simulink model "P_Like"  (Simulink 7.3)
settings: Solver=ode45  StartTime=0.0  StopTime=100  RelTol=1e-3
values from neighbouring files (symbols this model uses):
  Dm = 0.2    [Parameters.m]
  Ds = 0.1    [Parameters.m]
  K = ceil(max(K1,K2))    [Gains.m]
  Lm1 = 0.5    [Parameters.m]
  Lm2 = 0.5    [Parameters.m]
  Ls1 = 0.5    [Parameters.m]
  Ls2 = 0.5    [Parameters.m]
  Mm1 = 1    [Parameters.m]
  Mm2 = 1    [Parameters.m]
  Ms1 = 2    [Parameters.m]
  Ms2 = 2    [Parameters.m]
  P = 10    [Parameters.m]
  q0 = [0;0]    [Parameters.m]
  v0 = [0;0;0]    [Initiation.m]    (also in Parameters.m = [0;0])
settings Model: Creator=TOSHIBA  LastModifiedBy=TOSHIBA  CovModelRefEnable=off
settings DataIOCC: SaveFormat=StructureWithTime  ReturnWorkspaceOutputs=off
settings OptimizationCC: ExpressionDepthLimit=128
settings DebuggingCC: UnderspecifiedInitializationDetection=Simplified  MergeDetectMultiDrivingBlocksExec=error  SolverPrmCheckMsg=none  FcnCallInpInsideContextMsg=Enable All  StateNameClashWarn=none  StrictBusMsg=ErrorLevel1
settings HardwareCC: ProdIntDivRoundTo=Zero  ProdEndianess=LittleEndian  ProdHWDeviceType=Specified
settings CodeAppCC: CustomSymbolStrType=$N$R$M_T
settings GRTTargetCC: TargetFunctionLibrary=C89/C90 (ANSI)

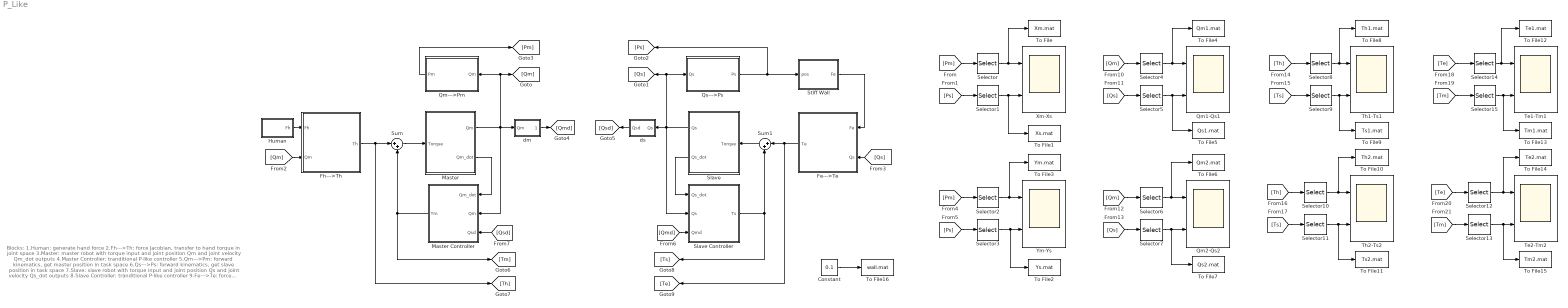
== system P_Like ==
  note: Blocks:
      | 1.Human: generate hand force
      | 2.Fh--->Th: force Jacobian, transfer to hand torque in joint space
      | 3.Master: master robot with torque input and joint position Qm and joint velocity Qm_dot outputs
      | 4.Master Controller: tranditional P-like controller
      | 5.Qm--->Pm: forward kinematics, get master position in task space
      | 6.Qs--->Ps: forward kinematics, get slave position in task space
      | 7.Slave: slave robot with torque input and joint position Qs and joint velocity Qs_dot outputs
      | 8.Slave Controller: tranditional P-like controller
      | 9.Fe--->Te: force Jacobian, transfer to environment torque in joint space
      | 10.Stiff Wall: spring with k=10KN/m
  Constant : Constant  Value=0.1
  Fe--->Te : Subsystem
  Fh--->Th : Subsystem
  Human : Subsystem
  Master : Subsystem
  Master Controller : Subsystem
  Qm--->Pm : Subsystem
  Qm1-Qs1 : Scope  NumInputPorts=2
      settings: TimeRange=auto  MaxDataPoints=5000  SaveToWorkspace=off  SaveName=ScopeData2  YMin=-0.1601~-5  YMax=0.25682~5  SampleTime=-1
  Qm2-Qs2 : Scope  NumInputPorts=2
      settings: TimeRange=auto  MaxDataPoints=5000  SaveToWorkspace=off  SaveName=ScopeData3  YMin=-0.08778~-5  YMax=0.12467~5  SampleTime=-1
  Qs--->Ps : Subsystem
  Selector{,1,4..5,8..9,14..15} (8 alike) : Selector  InputPortWidth=2  IndexOptions=Index vector (dialog)  Indices=[1]  OutputSizes=1
  Selector{2..3,6..7,10..13} (8 alike) : Selector  InputPortWidth=2  IndexOptions=Index vector (dialog)  Indices=[2]  OutputSizes=1
  Slave : Subsystem
  Slave Controller : Subsystem
  Stiff Wall : Stateflow chart  TreatAsAtomicUnit=on
      settings: PermitHierarchicalResolution=ParametersOnly
  Sum : Sum  Inputs=|++
  Sum1 : Sum  Inputs=|++
  Te1-Tm1 : Scope  NumInputPorts=2
      settings: TimeRange=auto  MaxDataPoints=5000  SaveToWorkspace=off  SaveName=ScopeData6  YMin=-10.54121~-5  YMax=1.73671~5  SampleTime=-1
  Te2-Tm2 : Scope  NumInputPorts=2
      settings: TimeRange=auto  MaxDataPoints=5000  SaveToWorkspace=off  SaveName=ScopeData7  YMin=-5.26164~-5  YMax=0.8676~5  SampleTime=-1
  Th1-Ts1 : Scope  NumInputPorts=2
      settings: TimeRange=auto  MaxDataPoints=5000  SaveToWorkspace=off  SaveName=ScopeData4  YMin=-0.80713~-5  YMax=2.31036~5  SampleTime=-1
  Th2-Ts2 : Scope  NumInputPorts=2
      settings: TimeRange=auto  MaxDataPoints=5000  SaveToWorkspace=off  SaveName=ScopeData5  YMin=-0.4004~-5  YMax=1.10559~5  SampleTime=-1
  To File : ToFile  Filename=Xm.mat  MatrixName=Xm
  To File1 : ToFile  Filename=Xs.mat  MatrixName=Xs
  To File10 : ToFile  Filename=Th2.mat  MatrixName=Th2
  To File11 : ToFile  Filename=Ts2.mat  MatrixName=Ts2
  To File12 : ToFile  Filename=Te1.mat  MatrixName=Te1
  To File13 : ToFile  Filename=Tm1.mat  MatrixName=Tm1
  To File14 : ToFile  Filename=Te2.mat  MatrixName=Te2
  To File15 : ToFile  Filename=Tm2.mat  MatrixName=Tm2
  To File16 : ToFile  Filename=wall.mat  MatrixName=wall
  To File2 : ToFile  Filename=Ys.mat  MatrixName=Ys
  To File3 : ToFile  Filename=Ym.mat  MatrixName=Ym
  To File4 : ToFile  Filename=Qm1.mat  MatrixName=Qm1
  To File5 : ToFile  Filename=Qs1.mat  MatrixName=Qs1
  To File6 : ToFile  Filename=Qm2.mat  MatrixName=Qm2
  To File7 : ToFile  Filename=Qs2.mat  MatrixName=Qs2
  To File8 : ToFile  Filename=Th1.mat  MatrixName=Th1
  To File9 : ToFile  Filename=Ts1.mat  MatrixName=Ts1
  Xm-Xs : Scope  NumInputPorts=2
      settings: TimeRange=auto  MaxDataPoints=5000  SaveToWorkspace=off  SaveName=ScopeData  YMin=0.95971~-5  YMax=1.00448~5  SampleTime=-1
  Ym-Ys : Scope  NumInputPorts=2
      settings: TimeRange=auto  MaxDataPoints=5000  SaveToWorkspace=off  YMin=-0.20079~-5  YMax=0.31146~5  SampleTime=-1
  dm : Subsystem
  ds : Subsystem
  wires:
  Qs--->Ps/1(Ps) -> [Ps], Stiff Wall/1(pos)
  Stiff Wall/1(Fe) -> Fe--->Te/1(Fe)
  Fe--->Te/1(Te) -> Sum1/1, [Te]
  Sum1/1 -> Slave/1(Torque)
  Sum/1 -> Master/1(Torque)
  Fh--->Th/1(Th) -> [Th], Sum/1
  Master/2(Qm_dot) -> Master Controller/1(Qm_dot)
  Master Controller/1(Tm) -> Sum/2, [Tm]
  Slave/2(Qs_dot) -> Slave Controller/1(Qs_dot)
  Slave Controller/1(Ts) -> [Ts], Sum1/2
  [Qs] -> Fe--->Te/2(Qs)
  Master/1(Qm) -> dm/1(Qm), Qm--->Pm/1(Qm), [Qm], Master Controller/2(Qm)
  Slave/1(Qs) -> ds/1(Qs), [Qs], Qs--->Ps/1(Qs), Slave Controller/2(Qs)
  [Qm] -> Fh--->Th/2(Qm)
  Human/1(Fh) -> Fh--->Th/1(Fh)
  Qm--->Pm/1(Pm) -> [Pm]
  [Pm] -> Selector/1
  Selector/1 -> To File/1, Xm-Xs/1
  [Ps] -> Selector1/1
  Selector1/1 -> To File1/1, Xm-Xs/2
  [Pm] -> Selector2/1
  Selector2/1 -> To File3/1, Ym-Ys/1
  [Ps] -> Selector3/1
  Selector3/1 -> To File2/1, Ym-Ys/2
  [Qmd] -> Slave Controller/3(Qmd)
  dm/1(Qmd) -> [Qmd]
  ds/1(Qsd) -> [Qsd]
  [Qsd] -> Master Controller/3(Qsd)
  [Qs] -> Selector5/1
  [Qm] -> Selector4/1
  Selector4/1 -> To File4/1, Qm1-Qs1/1
  Selector5/1 -> To File5/1, Qm1-Qs1/2
  [Qs] -> Selector7/1
  [Qm] -> Selector6/1
  Selector6/1 -> To File6/1, Qm2-Qs2/1
  Selector7/1 -> To File7/1, Qm2-Qs2/2
  [Th] -> Selector8/1
  [Ts] -> Selector9/1
  Selector9/1 -> To File9/1, Th1-Ts1/2
  Selector8/1 -> To File8/1, Th1-Ts1/1
  [Ts] -> Selector11/1
  [Th] -> Selector10/1
  Selector10/1 -> To File10/1, Th2-Ts2/1
  [Te] -> Selector14/1
  [Tm] -> Selector15/1
  Selector15/1 -> To File13/1, Te1-Tm1/2
  Selector14/1 -> To File12/1, Te1-Tm1/1
  [Tm] -> Selector13/1
  [Te] -> Selector12/1
  Selector12/1 -> To File14/1, Te2-Tm2/1
  Selector13/1 -> To File15/1, Te2-Tm2/2
  Selector11/1 -> To File11/1, Th2-Ts2/2
  Constant/1 -> To File16/1

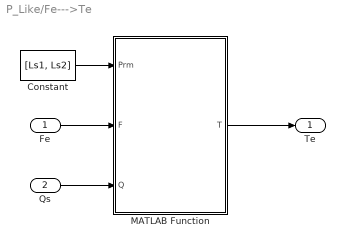
== system P_Like/Fe--->Te ==
  Fe : Inport
  Qs : Inport  Port=2
  Constant : Constant  Value=[Ls1, Ls2]
  MATLAB Function : Stateflow chart  TreatAsAtomicUnit=on
      settings: PermitHierarchicalResolution=ParametersOnly
  Te : Outport
  wires:
  Qs/1 -> MATLAB Function/3(Q)
  Fe/1 -> MATLAB Function/2(F)
  MATLAB Function/1(T) -> Te/1
  Constant/1 -> MATLAB Function/1(Prm)

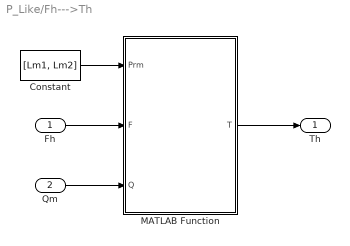
== system P_Like/Fh--->Th ==
  Fh : Inport
  Qm : Inport  Port=2
  Constant : Constant  Value=[Lm1, Lm2]
  MATLAB Function : Stateflow chart  TreatAsAtomicUnit=on
      settings: PermitHierarchicalResolution=ParametersOnly
  Th : Outport
  wires:
  Fh/1 -> MATLAB Function/2(F)
  MATLAB Function/1(T) -> Th/1
  Qm/1 -> MATLAB Function/3(Q)
  Constant/1 -> MATLAB Function/1(Prm)

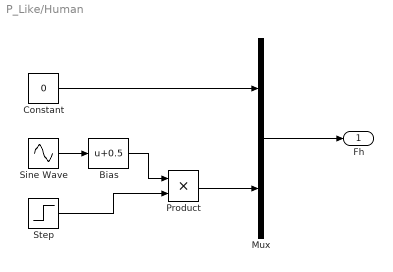
== system P_Like/Human ==
  Bias : Bias  Bias=0.5
  Constant : Constant  Value=0
  Mux : Mux  Inputs=2
  Product : Product
  Sine Wave : Sin  Frequency=pi/20  SampleTime=0
  Step : Step  Time=100  Before=1  After=0  SampleTime=0
  Fh : Outport
  wires:
  Mux/1 -> Fh/1
  Constant/1 -> Mux/1
  Step/1 -> Product/2
  Bias/1 -> Product/1
  Product/1 -> Mux/2
  Sine Wave/1 -> Bias/1

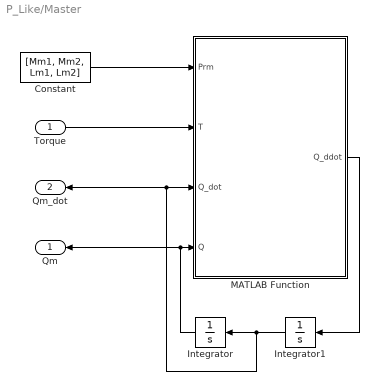
== system P_Like/Master ==
  Torque : Inport
  Constant : Constant  Value=[Mm1, Mm2, Lm1, Lm2]
  Integrator : Integrator  InitialCondition=q0
  Integrator1 : Integrator  InitialCondition=v0
  MATLAB Function : Stateflow chart  TreatAsAtomicUnit=on
      settings: PermitHierarchicalResolution=ParametersOnly
  Qm : Outport
  Qm_dot : Outport  Port=2
  wires:
  Torque/1 -> MATLAB Function/2(T)
  Constant/1 -> MATLAB Function/1(Prm)
  MATLAB Function/1(Q_ddot) -> Integrator1/1
  Integrator1/1 -> Qm_dot/1, MATLAB Function/3(Q_dot), Integrator/1
  Integrator/1 -> Qm/1, MATLAB Function/4(Q)

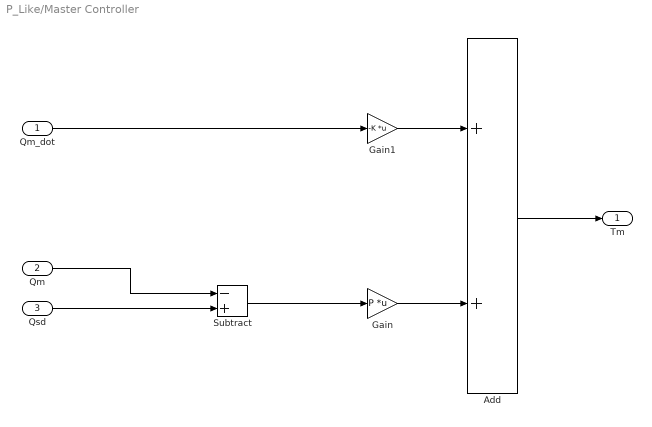
== system P_Like/Master Controller ==
  Qm_dot : Inport
  Qm : Inport  Port=2
  Qsd : Inport  Port=3
  Add : Sum
  Gain : Gain  Gain=P  Multiplication=Matrix(K*u) (u vector)
  Gain1 : Gain  Gain=-K  Multiplication=Matrix(K*u) (u vector)
  Subtract : Sum  Inputs=-+
  Tm : Outport
  wires:
  Qm/1 -> Subtract/1
  Qsd/1 -> Subtract/2
  Gain/1 -> Add/2
  Gain1/1 -> Add/1
  Add/1 -> Tm/1
  Qm_dot/1 -> Gain1/1
  Subtract/1 -> Gain/1

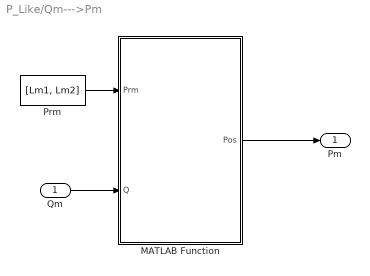
== system P_Like/Qm--->Pm ==
  Qm : Inport
  MATLAB Function : Stateflow chart  TreatAsAtomicUnit=on
      settings: PermitHierarchicalResolution=ParametersOnly
  Prm : Constant  Value=[Lm1, Lm2]
  Pm : Outport
  wires:
  MATLAB Function/1(Pos) -> Pm/1
  Qm/1 -> MATLAB Function/2(Q)
  Prm/1 -> MATLAB Function/1(Prm)

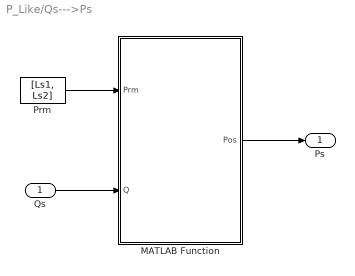
== system P_Like/Qs--->Ps ==
  Qs : Inport
  MATLAB Function : Stateflow chart  TreatAsAtomicUnit=on
      settings: PermitHierarchicalResolution=ParametersOnly
  Prm : Constant  Value=[Ls1, Ls2]
  Ps : Outport
  wires:
  Qs/1 -> MATLAB Function/2(Q)
  MATLAB Function/1(Pos) -> Ps/1
  Prm/1 -> MATLAB Function/1(Prm)

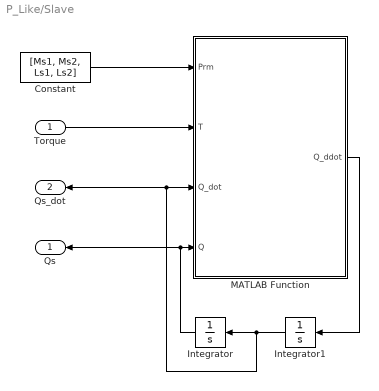
== system P_Like/Slave ==
  Torque : Inport
  Constant : Constant  Value=[Ms1, Ms2, Ls1, Ls2]
  Integrator : Integrator  InitialCondition=q0
  Integrator1 : Integrator  InitialCondition=v0
  MATLAB Function : Stateflow chart  TreatAsAtomicUnit=on
      settings: PermitHierarchicalResolution=ParametersOnly
  Qs : Outport
  Qs_dot : Outport  Port=2
  wires:
  Torque/1 -> MATLAB Function/2(T)
  Constant/1 -> MATLAB Function/1(Prm)
  MATLAB Function/1(Q_ddot) -> Integrator1/1
  Integrator1/1 -> Qs_dot/1, MATLAB Function/3(Q_dot), Integrator/1
  Integrator/1 -> Qs/1, MATLAB Function/4(Q)

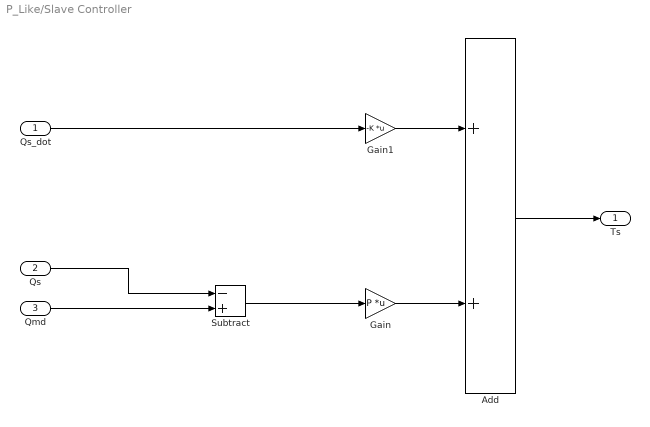
== system P_Like/Slave Controller ==
  Qs_dot : Inport
  Qs : Inport  Port=2
  Qmd : Inport  Port=3
  Add : Sum
  Gain : Gain  Gain=P  Multiplication=Matrix(K*u) (u vector)
  Gain1 : Gain  Gain=-K  Multiplication=Matrix(K*u) (u vector)
  Subtract : Sum  Inputs=-+
  Ts : Outport
  wires:
  Subtract/1 -> Gain/1
  Qs_dot/1 -> Gain1/1
  Add/1 -> Ts/1
  Gain1/1 -> Add/1
  Gain/1 -> Add/2
  Qmd/1 -> Subtract/2
  Qs/1 -> Subtract/1

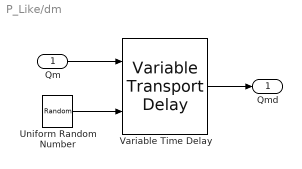
== system P_Like/dm ==
  Qm : Inport
  Uniform Random Number : UniformRandomNumber  Minimum=0  Maximum=Dm  SampleTime=0.1
  Variable Time Delay : VariableTransportDelay  MaximumDelay=Dm
  Qmd : Outport
  wires:
  Qm/1 -> Variable Time Delay/1
  Uniform Random Number/1 -> Variable Time Delay/2
  Variable Time Delay/1 -> Qmd/1

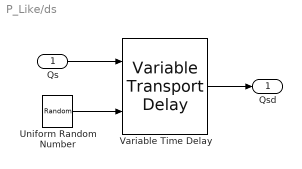
== system P_Like/ds ==
  Qs : Inport
  Uniform Random Number : UniformRandomNumber  Minimum=0  Maximum=Ds  SampleTime=0.1
  Variable Time Delay : VariableTransportDelay  MaximumDelay=Ds
  Qsd : Outport
  wires:
  Uniform Random Number/1 -> Variable Time Delay/2
  Qs/1 -> Variable Time Delay/1
  Variable Time Delay/1 -> Qsd/1

== matlab function Master/MATLAB Function ==
  data: Prm input double; Q_ddot output double; T input double; Q_dot input double; Q input double
function Q_ddot  = RobotArm_2DOF(Prm, T, Q_dot, Q)
%#eml
g = 9.8;
m1 = Prm(1);
m2 = Prm(2);
l1 = Prm(3);
l2 = Prm(4);
q1 = Q(1);
q2 = Q(2);
q1_dot = Q_dot(1);
q2_dot = Q_dot(2);
M11 = m2*l2^2+(m1+m2)*l1^2+2*m2*l1*l2*cos(q2);
M12 = m2*l2^2+m2*l1*l2*cos(q2);
M21 = M12;
M22 = m2*l2^2;
M = [M11, M12; M21, M22];
C11 = -2*m2*l1*l2*sin(q2)*q2_dot;
C12 = -m2*l1*l2*sin(q2)*q2_dot;
C21 = m2*l1*l2*sin(q2)*q1_dot;
C22 = 0;
C = [C11, C12; C21, C22];
g1 = m2*g*l2*sin(q1+q2)+(m1+m2)*g*l1*sin(q1);
g2 = m2*g*l2*sin(q1+q2);
G = [g1; g2];
Q_ddot = M\(T-C*Q_dot);

== matlab function Stiff Wall ==
  data: pos input double; Fe output double
function Fe  = Envir(pos)
%#eml
kWall = 10000;
if pos(2)>=0.1
    Fe=[0; -(pos(2)-0.1)*kWall];
    if Fe(2)>0
        Fe = zeros(2,1);
    end
else
    Fe=zeros(2,1);
end

== matlab function Slave/MATLAB Function ==
  data: Prm input double; Q_ddot output double; T input double; Q_dot input double; Q input double
function Q_ddot  = RobotArm_2DOF(Prm, T, Q_dot, Q)
%#eml
g = 9.8;
m1 = Prm(1);
m2 = Prm(2);
l1 = Prm(3);
l2 = Prm(4);
q1 = Q(1);
q2 = Q(2);
q1_dot = Q_dot(1);
q2_dot = Q_dot(2);
M11 = m2*l2^2+(m1+m2)*l1^2+2*m2*l1*l2*cos(q2);
M12 = m2*l2^2+m2*l1*l2*cos(q2);
M21 = M12;
M22 = m2*l2^2;
M = [M11, M12; M21, M22];
C11 = -2*m2*l1*l2*sin(q2)*q2_dot;
C12 = -m2*l1*l2*sin(q2)*q2_dot;
C21 = m2*l1*l2*sin(q2)*q1_dot;
C22 = 0;
C = [C11, C12; C21, C22];
g1 = m2*g*l2*sin(q1+q2)+(m1+m2)*l1*sin(q1);
g2 = m2*g*l2*sin(q1+q2);
G = [g1; g2];
Q_ddot = M\(T-C*Q_dot);

== matlab function Qm--->Pm/MATLAB Function ==
  data: Prm input double; Pos output double; Q input double
function Pos = ForwardKinematics(Prm, Q)
%#eml
l1 = Prm(1);
l2 = Prm(2);
q1 = Q(1);
q2 = Q(2);
x = l1*cos(q1)+l2*cos(q1+q2);
y = l1*sin(q1)+l2*sin(q1+q2);
Pos = [x; y];

== matlab function Qs--->Ps/MATLAB Function ==
  data: Prm input double; Pos output double; Q input double
function Pos = ForwardKinematics(Prm, Q)
%#eml
l1 = Prm(1);
l2 = Prm(2);
q1 = Q(1);
q2 = Q(2);
x = l1*cos(q1)+l2*cos(q1+q2);
y = l1*sin(q1)+l2*sin(q1+q2);
Pos = [x; y];

== matlab function Fh--->Th/MATLAB Function ==
  data: Prm input double; T output double; F input double; Q input double
function T = Force_to_Torque(Prm, F, Q)
%#eml
l1 = Prm(1);
l2 = Prm(2);
q1 = Q(1);
q2 = Q(2);
J11 = -l1*sin(q1)-l2*sin(q1+q2);
J12 = -l2*sin(q1+q2);
J21 = l1*cos(q1)+l2*cos(q1+q2);
J22 = l2*cos(q1+q2);
J = [J11, J12; J21, J22];
T = J'*F;

== matlab function Fe--->Te/MATLAB Function ==
  data: Prm input double; T output double; F input double; Q input double
function T = Force_to_Torque(Prm, F, Q)
%#eml
l1 = Prm(1);
l2 = Prm(2);
q1 = Q(1);
q2 = Q(2);
J11 = -l1*sin(q1)-l2*sin(q1+q2);
J12 = -l2*sin(q1+q2);
J21 = l1*cos(q1)+l2*cos(q1+q2);
J22 = l2*cos(q1+q2);
J = [J11, J12; J21, J22];
T = J'*F;
